simulink model "SimulinkP7_2"  (R2018b)
settings: Solver=VariableStepAuto  StartTime=0.0  StopTime=10.0  RelTol=1e-3
values from neighbouring files (symbols this model uses):
  A = [  0  1; -2 -3 ]    [problema7_2.m]
  B = [ 0; 4]    [problema7_2.m]
  C = [ 1 0 ]    [problema7_2.m]
  C1 = [ 0 1 ]    [problema7_2.m]
  Ca = [1 0; 0 1]    [problema7_2.m]
  D = 0    [problema7_2.m]
  Da = [0; 0]    [problema7_2.m]
  h = 0.1    [problema7_2.m]
  L = [0 1] * inv(Wc) * (phi^2 + p1 * phi + p2 * eye(2))    [problema7_2.m]
  Lc = 1/( C * inv(eye(2) - phic ) * gama )    [problema7_2.m]
settings Model: Creator=fredericovaz  LastModifiedBy=fredericovaz

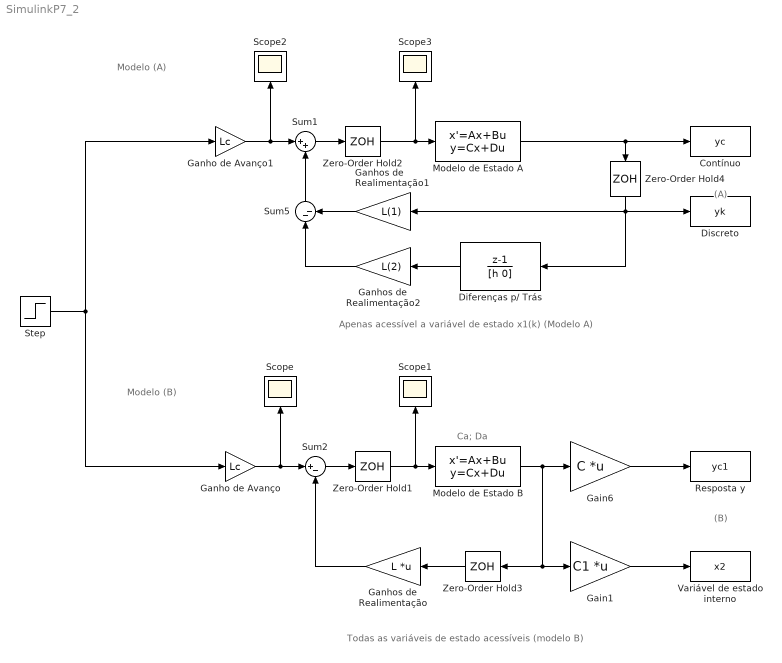
== system SimulinkP7_2 ==
  note: Ca; Da
  note: Apenas acessível a variável de estado x1(k) (Modelo A)
  note: (A)
  note: Modelo (B)
  note: (B)
  note: Modelo (A)
  note: Todas as variáveis de estado acessíveis (modelo B)
  Contínuo : ToWorkspace  VariableName=yc  SaveFormat=Structure With Time  SampleTime=-1
  Diferenças p/ Trás : DiscreteTransferFcn  Numerator=[1 -1]  Denominator=[h 0]
  Discreto : ToWorkspace  VariableName=yk  SaveFormat=Structure With Time  SampleTime=-1
  Gain1 : Gain  Gain=C1  Multiplication=Matrix(K*u) (u vector)
  Gain6 : Gain  Gain=C  Multiplication=Matrix(K*u) (u vector)
  Ganho de Avanço : Gain  Gain=Lc
  Ganho de Avanço1 : Gain  Gain=Lc
  Ganhos de Realimentação : Gain  Gain=L  Multiplication=Matrix(K*u) (u vector)
  Ganhos de Realimentação1 : Gain  Gain=L(1)
  Ganhos de Realimentação2 : Gain  Gain=L(2)
  Modelo de Estado A : StateSpace  A=A  B=B  C=C  D=D  InitialCondition=0
  Modelo de Estado B : StateSpace  A=A  B=B  C=Ca  D=Da  InitialCondition=0
  Resposta y : ToWorkspace  VariableName=yc1  SaveFormat=Structure With Time  SampleTime=-1
  Scope{,1..3} (4 alike) : Scope
  Step : Step  Time=0  SampleTime=0
  Sum1 : Sum  Inputs=|++
  Sum2 : Sum  Inputs=|+-
  Sum5 : Sum  Inputs=|--
  Variável de estado interno : ToWorkspace  VariableName=x2  SaveFormat=Structure With Time  SampleTime=-1
  Zero-Order Hold{1..4} (4 alike) : ZeroOrderHold  SampleTime=h
  wires:
  Modelo de Estado B/1 -> Zero-Order Hold3/1, Gain1/1, Gain6/1
  Sum5/1 -> Sum1/2
  Gain6/1 -> Resposta y/1
  Gain1/1 -> Variável de estado interno/1
  Ganho de Avanço1/1 -> Sum1/1, Scope2/1
  Ganho de Avanço/1 -> Sum2/1, Scope/1
  Ganhos de Realimentação1/1 -> Sum5/2
  Zero-Order Hold4/1 -> Ganhos de Realimentação1/1, Diferenças p/ Trás/1, Discreto/1
  Modelo de Estado A/1 -> Contínuo/1, Zero-Order Hold4/1
  Ganhos de Realimentação/1 -> Sum2/2
  Diferenças p/ Trás/1 -> Ganhos de Realimentação2/1
  Sum2/1 -> Zero-Order Hold1/1
  Zero-Order Hold2/1 -> Scope3/1, Modelo de Estado A/1
  Zero-Order Hold1/1 -> Scope1/1, Modelo de Estado B/1
  Ganhos de Realimentação2/1 -> Sum5/1
  Sum1/1 -> Zero-Order Hold2/1
  Step/1 -> Ganho de Avanço/1, Ganho de Avanço1/1
  Zero-Order Hold3/1 -> Ganhos de Realimentação/1
